simulink library "BRPI_lib"  (Simulink 7.5)
settings: Solver=ode45  StartTime=0.0  StopTime=10.0  RelTol=1e-3
values from neighbouring files (symbols this model uses):
  pBRPI_bar_BrkPedSwtThrsh_C = Simulink.Parameter    [BRPI_par.m]
  pBRPI_bar_BrkPresSubHi_C = Simulink.Parameter    [BRPI_par.m]
  pBRPI_bar_BrkPresSubLo_C = Simulink.Parameter    [BRPI_par.m]
  pBRPI_s_BrkPedlPsdChkTiout_C = Simulink.Parameter    [BRPI_par.m]
undefined symbols (not defined in the file or in its folder): DiscIntNeverNeededParam, p_bool_True_M
libraries: BaseOperationLib_Browser x14, PES_CZ_FAW x2, simulink x1
settings Model: Creator=wuaibin  LastModifiedBy=wuaibin

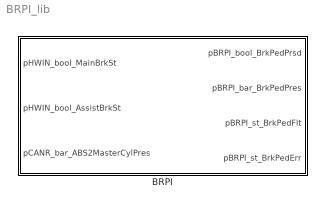
== system BRPI_lib ==
  BRPI : Subsystem  TreatAsAtomicUnit=on

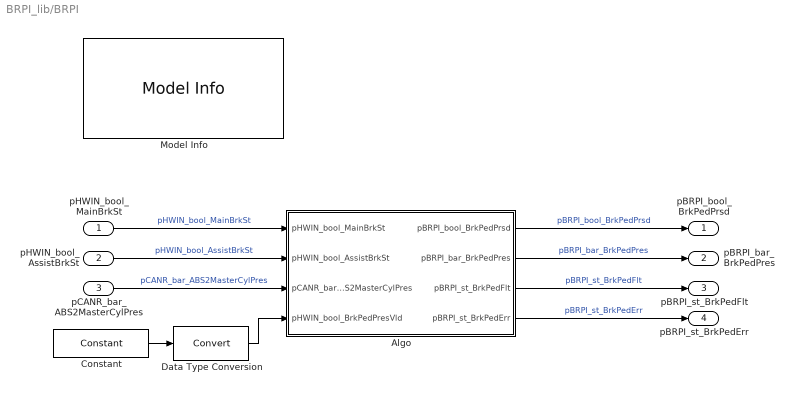
== system BRPI_lib/BRPI ==
  pHWIN_bool_MainBrkSt : Inport  OutDataType=fixdt(1, 16)  OutScaling=2^0
  pHWIN_bool_AssistBrkSt : Inport  Port=2  OutDataType=fixdt(1, 16)  OutScaling=2^0
  pCANR_bar_ABS2MasterCylPres : Inport  Port=3  OutDataType=fixdt(1, 16)  OutScaling=2^0
  Algo : Subsystem
  Constant : BaseOperationLib_Browser/Sources&Sinks/Constant  Value=p_bool_True_M  OutMin=[]  OutMax=[]  OutDataType=fixdt(1, 16)  ConRadixGroup=Use specified scaling  OutScaling=2^0  OutDataTypeStr=Inherit: Inherit via back propagation
  Data Type Conversion : DataTypeConversion  OutDataType=fixdt(1, 16)  OutScaling=2^0
  Model Info : simulink/Model-Wide Utilities/Model Info  SystemSampleTime=-1  InitialBlockCM=None  BlockCM=None  Frame=on  DisplayStringWithTags=Model Info\nCreated: %<Created>\nCreator: %<Creator>  HorizontalTextAlignment=Center  LeftAlignmentValue=0.5  SourceBlockDiagram=HQEV_HCU  TagMaxNumber=20
  pBRPI_bool_BrkPedPrsd : Outport  OutDataType=fixdt(1, 16)  OutScaling=2^0
  pBRPI_bar_BrkPedPres : Outport  Port=2  OutDataType=fixdt(1, 16)  OutScaling=2^0
  pBRPI_st_BrkPedFlt : Outport  Port=3  OutDataType=fixdt(1, 16)  OutScaling=2^0
  pBRPI_st_BrkPedErr : Outport  Port=4  OutDataType=fixdt(1, 16)  OutScaling=2^0
  wires:
  Constant/1 -> Data Type Conversion/1
  Data Type Conversion/1 -> Algo/4(pHWIN_bool_BrkPedPresVld)
  Algo/4(pBRPI_st_BrkPedErr) -> pBRPI_st_BrkPedErr/1  "pBRPI_st_BrkPedErr"
  pCANR_bar_ABS2MasterCylPres/1 -> Algo/3(pCANR_bar_ABS2MasterCylPres)  "pCANR_bar_ABS2MasterCylPres"
  Algo/3(pBRPI_st_BrkPedFlt) -> pBRPI_st_BrkPedFlt/1  "pBRPI_st_BrkPedFlt"
  Algo/2(pBRPI_bar_BrkPedPres) -> pBRPI_bar_BrkPedPres/1  "pBRPI_bar_BrkPedPres"
  Algo/1(pBRPI_bool_BrkPedPrsd) -> pBRPI_bool_BrkPedPrsd/1  "pBRPI_bool_BrkPedPrsd"
  pHWIN_bool_AssistBrkSt/1 -> Algo/2(pHWIN_bool_AssistBrkSt)  "pHWIN_bool_AssistBrkSt"
  pHWIN_bool_MainBrkSt/1 -> Algo/1(pHWIN_bool_MainBrkSt)  "pHWIN_bool_MainBrkSt"

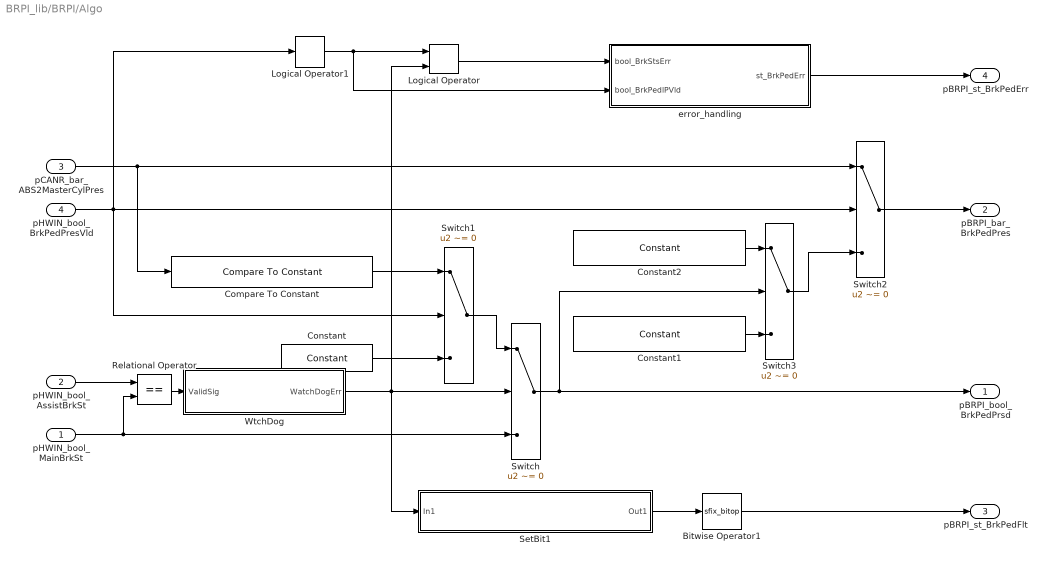
== system BRPI_lib/BRPI/Algo ==
  pHWIN_bool_MainBrkSt : Inport  OutDataType=fixdt(1, 16)  OutScaling=2^0
  pHWIN_bool_AssistBrkSt : Inport  Port=2  OutDataType=fixdt(1, 16)  OutScaling=2^0
  pCANR_bar_ABS2MasterCylPres : Inport  Port=3  OutDataType=fixdt(1, 16)  OutScaling=2^0
  pHWIN_bool_BrkPedPresVld : Inport  Port=4  OutDataType=fixdt(1, 16)  OutScaling=2^0
  Bitwise Operator1 : S-Function  FunctionName=sfix_bitop  Parameters=UseBitMask,NumInputPorts,BitMask,BitMaskRealWorld,logicop  EnableBusSupport=off  mask(Bitwise Operator){logicop=OR, UseBitMask=off, NumInputPorts=1, BitMask=bin2dec('11011001'), BitMaskRealWorld=Stored Integer}
      mask prompts: logicop "Operator:"; UseBitMask "Use bit mask ..."; NumInputPorts "Number of input ports:"; BitMask "Bit Mask"; BitMaskRealWorld "Treat mask as:"
      mask help: Perform the specified bitwise operation on the inputs. The output data type should represent zero exactly.
      mask init:
      | str = '';
      | if UseBitMask
      |   [m,n] = size(BitMask);
      |   if ischar(BitMask)
      |     len = m;
      |     n = 1;
      |   else
      |     len = m * n;
      |   end
      |   internalBitMask = zeros(m,n);
      |   if isnumeric(BitMask)
      |     for i=1:len,
      |       internalBitMask(i) = BitMask(i);
      |     end
      |   elseif ischar(BitMask)
      |     for i=1:m,
      |       internalBitMask(i) = hex2dec(BitMask(i,:));
      |     end
      |   elseif iscell(BitMask)
      |     for i=1:len,
      |       if isnumeric( BitMask{i} )
      |         internalBitMask(i) = BitMask{i};
      |       elseif ischar( BitMask{i} )
      |         internalBitMask(i) = hex2dec(BitMask{i});
      |       else
      |         errordlg(['Data type is not supported at cell item ', num2str(i) ]);
      |       end
      |     end
      |   end
      |   BitMask = internalBitMask;
      |   for i=1:len
      |     if BitMask(i) > (2^52)-1
      |       error(DAStudio.message('Simulink:blocks:BitMaskWordLengthTooLarge')); 
      |     end
      |   end 
      |   if len == 1
      |      if BitMaskRealWorld == 1 || BitMask(1) < 0
      |        str=num2str(BitMask(1));
      |      else
      |        str=['0x',dec2hex(floor(BitMask(1)))];
      |      end
      |   else
      |      str='Masks';
      |   end
      | else
      |   BitMask = 0;
      |   str='';
      | end
      mask StyleString: popup(AND|OR|NAND|NOR|XOR|NOT),checkbox,edit,edit,popup(Real World Value|Stored Integer)
      mask CallbackString: fixptdialog(gcbh)|fixptdialog(gcbh)|||
      mask Display: fprintf(['Bitwise\n',logicop,'\n',str])
  Compare To Constant : BaseOperationLib_Browser/Logic Operations Changed/Compare To Constant  SystemSampleTime=-1  relop=>=  const=pBRPI_bar_BrkPedSwtThrsh_C
  Constant : BaseOperationLib_Browser/Sources&Sinks/Constant  Value=p_bool_True_M  OutMin=[]  OutMax=[]  OutDataType=fixdt(1, 16)  ConRadixGroup=Use specified scaling  OutScaling=2^0  OutDataTypeStr=Inherit: Inherit via back propagation
  Constant1 : BaseOperationLib_Browser/Sources&Sinks/Constant  Value=pBRPI_bar_BrkPresSubLo_C  OutMin=[]  OutMax=[]  OutDataType=fixdt(1, 16)  ConRadixGroup=Use specified scaling  OutScaling=2^0  OutDataTypeStr=Inherit: Inherit via back propagation
  Constant2 : BaseOperationLib_Browser/Sources&Sinks/Constant  Value=pBRPI_bar_BrkPresSubHi_C  OutMin=[]  OutMax=[]  OutDataType=fixdt(1, 16)  ConRadixGroup=Use specified scaling  OutScaling=2^0  OutDataTypeStr=Inherit: Inherit via back propagation
  Logical Operator : BaseOperationLib_Browser/Logic Operations Changed/Logical Operator  Operator=AND  Inputs=2  AllPortsSameDT=on  OutDataTypeMode=Specify via dialog  LogicDataType=PDT_Bool  OutDataTypeStr=PDT_Bool
  Logical Operator1 : BaseOperationLib_Browser/Logic Operations Changed/Logical Operator  Operator=NOT  Inputs=2  AllPortsSameDT=on  OutDataTypeMode=Specify via dialog  LogicDataType=PDT_Bool  OutDataTypeStr=PDT_Bool
  Relational Operator : RelationalOperator  Operator===  LogicOutDataTypeMode=Specify via dialog  LogicDataType=PDT_Bool  OutDataTypeStr=PDT_Bool  InputSameDT=on
      mask Display: patch([0 1 1 1 .75], [1 1 0 .75 1], [0 1 0]);
  SetBit1 : Subsystem  mask{maska=BrkPedlFltTyp.BRAKE_PLAUSIBILITY_ERROR}
      mask prompts: maska "Set to value"
      mask help:
      | Set Bit
      |
      | Sets the bit specified by value if the input is greater than zero.
      |
      | Block is useful for encoding bit-encoded data.
      |
      | "Set to value" may not be a calibratable parameter.
      mask Help:
      | Set Bit
      | 
      | Sets the bit specified by value if the input is greater than zero.
      | 
      | Block is useful for encoding bit-encoded data.
      | 
      | "Set to value" may not be a calibratable parameter.
      mask Display: disp(['SetBit \n',maska]);
  Switch{,1..3} (4 alike) : Switch  Criteria=u2 ~= 0  Threshold=1  SaturateOnIntegerOverflow=on  InputSameDT=on
      mask Display: patch([0 1 1 1 .75], [1 1 0 .75 1], [0 1 0]);
  WtchDog : Subsystem  mask{timeoutthres=pBRPI_s_BrkPedlPsdChkTiout_C}
      mask prompts: timeoutthres "Timeout counter Treshold"
      mask help:
      | WatchDog block
      |
      | If input bool signal is false for the number of step bigger than "Timeout counter Threshold" the output WatchDog signal is set to True.
      |
      | Tip. Set the thresshold to the required time in seconds devided by algorithm sampling time.
      mask Help:
      | WatchDog block
      | 
      | If input bool signal is false for the number of step bigger than "Timeout counter Threshold" the output WatchDog signal is set to True.
      | 
      | Tip. Set the thresshold to required time in second devided by sampling time.
  error_handling : Subsystem
  pBRPI_bool_BrkPedPrsd : Outport  OutDataType=fixdt(1, 16)  OutScaling=2^0
  pBRPI_bar_BrkPedPres : Outport  Port=2  OutDataType=fixdt(1, 16)  OutScaling=2^0
  pBRPI_st_BrkPedFlt : Outport  Port=3  OutDataType=fixdt(1, 16)  OutScaling=2^0
  pBRPI_st_BrkPedErr : Outport  Port=4  OutDataType=fixdt(1, 16)  OutScaling=2^0
  wires:
  Bitwise Operator1/1 -> pBRPI_st_BrkPedFlt/1
  SetBit1/1(Out1) -> Bitwise Operator1/1
  Constant/1 -> Switch1/3
  Logical Operator/1 -> error_handling/1(bool_BrkStsErr)
  Logical Operator1/1 -> Logical Operator/1, error_handling/2(bool_BrkPedlPVld)
  Compare To Constant/1 -> Switch1/1
  Switch1/1 -> Switch/1
  error_handling/1(st_BrkPedErr) -> pBRPI_st_BrkPedErr/1
  pCANR_bar_ABS2MasterCylPres/1 -> Compare To Constant/1, Switch2/1
  pHWIN_bool_BrkPedPresVld/1 -> Logical Operator1/1, Switch1/2, Switch2/2
  WtchDog/1(WatchDogErr) -> SetBit1/1(In1), Logical Operator/2, Switch/2
  Relational Operator/1 -> WtchDog/1(ValidSig)
  Switch/1 -> pBRPI_bool_BrkPedPrsd/1, Switch3/2
  pHWIN_bool_AssistBrkSt/1 -> Relational Operator/1
  pHWIN_bool_MainBrkSt/1 -> Relational Operator/2, Switch/3
  Constant1/1 -> Switch3/3
  Constant2/1 -> Switch3/1
  Switch2/1 -> pBRPI_bar_BrkPedPres/1
  Switch3/1 -> Switch2/3

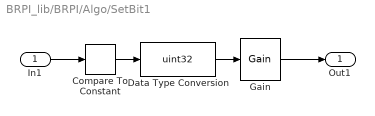
== system BRPI_lib/BRPI/Algo/SetBit1 ==
  In1 : Inport  OutDataType=fixdt(1, 16)  OutScaling=2^0
  Compare To Constant : BaseOperationLib_Browser/Logic Operations Changed/Compare To Constant  SystemSampleTime=-1  relop=>  const=0
  Data Type Conversion : DataTypeConversion  OutDataTypeMode=uint32  OutDataType=fixdt(1, 16)  OutScaling=2^0  OutDataTypeStr=uint32
  Gain : BaseOperationLib_Browser/Math Operations Changed/Gain  Gain=uint32(eval(maska))  Multiplication=Element-wise(K.*u)  ParamMin=[]  ParamMax=[]  ParameterDataType=fixdt(1, 16)  ParameterScalingMode=Best Precision: Matrix-wise  ParameterScaling=2^0  ParamDataTypeStr=Inherit: Inherit from 'Gain'  OutMin=[]  OutMax=[]  OutDataType=fixdt(1, 16)  OutScaling=2^0  SaturateOnIntegerOverflow=on
  Out1 : Outport  OutDataType=fixdt(1, 16)  OutScaling=2^0
  wires:
  Data Type Conversion/1 -> Gain/1
  In1/1 -> Compare To Constant/1
  Gain/1 -> Out1/1
  Compare To Constant/1 -> Data Type Conversion/1

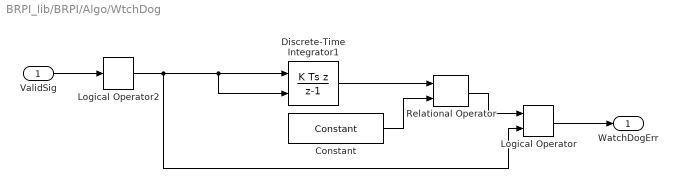
== system BRPI_lib/BRPI/Algo/WtchDog ==
  ValidSig : Inport  OutDataType=fixdt(1, 16)  OutScaling=2^0
  Constant : BaseOperationLib_Browser/Sources&Sinks/Constant  Value=timeoutthres  OutMin=[]  OutMax=[]  OutDataType=fixdt(1, 16)  ConRadixGroup=Use specified scaling  OutScaling=2^0  OutDataTypeStr=Inherit: Inherit from 'Constant value'
  Discrete-Time Integrator1 : DiscreteIntegrator  IntegratorMethod=Integration: Backward Euler  ExternalReset=rising  SampleTime=-1  OutDataType=PDT_s  OutDataTypeStr=Inherit: Inherit via back propagation  UpperSaturationLimit=100  LowerSaturationLimit=0  ICPrevOutput=DiscIntNeverNeededParam  ICPrevScaledInput=DiscIntNeverNeededParam
  Logical Operator : BaseOperationLib_Browser/Logic Operations Changed/Logical Operator  Operator=AND  Inputs=2  AllPortsSameDT=on  OutDataTypeMode=Specify via dialog  LogicDataType=PDT_Bool  OutDataTypeStr=PDT_Bool
  Logical Operator2 : BaseOperationLib_Browser/Logic Operations Changed/Logical Operator  Operator=NOT  Inputs=2  AllPortsSameDT=on  OutDataTypeMode=Specify via dialog  LogicDataType=PDT_Bool  OutDataTypeStr=PDT_Bool
  Relational Operator : BaseOperationLib_Browser/Logic Operations Changed/Relational Operator  Operator=>=  InputSameDT=on  LogicOutDataTypeMode=Specify via dialog  LogicDataType=PDT_Bool  OutDataTypeStr=PDT_Bool
  WatchDogErr : Outport  OutDataType=fixdt(1, 16)  OutScaling=2^0
  wires:
  Logical Operator2/1 -> Logical Operator/2, Discrete-Time Integrator1/2, Discrete-Time Integrator1/1
  Discrete-Time Integrator1/1 -> Relational Operator/1
  Constant/1 -> Relational Operator/2
  Logical Operator/1 -> WatchDogErr/1
  Relational Operator/1 -> Logical Operator/1
  ValidSig/1 -> Logical Operator2/1

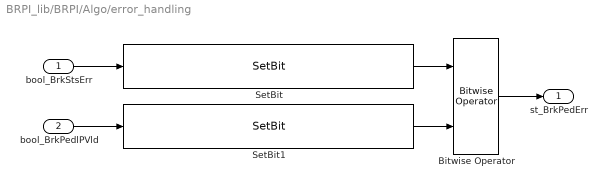
== system BRPI_lib/BRPI/Algo/error_handling ==
  bool_BrkStsErr : Inport
  bool_BrkPedlPVld : Inport  Port=2
  Bitwise Operator : BaseOperationLib_Browser/Others Unchanged/Bitwise Operator  logicop=OR  UseBitMask=off  NumInputPorts=2  BitMask=bin2dec('11011001')  BitMaskRealWorld=Stored Integer
  SetBit : PES_CZ_FAW/Discontinuities/SetBit  SystemSampleTime=-1  maska=FAWBrkPdlErrTyp.BRAKE_STATUS_ERROR
  SetBit1 : PES_CZ_FAW/Discontinuities/SetBit  SystemSampleTime=-1  maska=FAWBrkPdlErrTyp.BRAKE_PRESSURE_SIGNAL_ERROR
  st_BrkPedErr : Outport
  wires:
  SetBit1/1 -> Bitwise Operator/2
  SetBit/1 -> Bitwise Operator/1
  bool_BrkPedlPVld/1 -> SetBit1/1
  bool_BrkStsErr/1 -> SetBit/1
  Bitwise Operator/1 -> st_BrkPedErr/1
